simulink model "sx"  (R2015b)
settings: Solver=VariableStepAuto  StartTime=0.0  StopTime=0.003  RelTol=1e-3
settings Model: Creator=hohotulca  LastModifiedBy=hohotulca

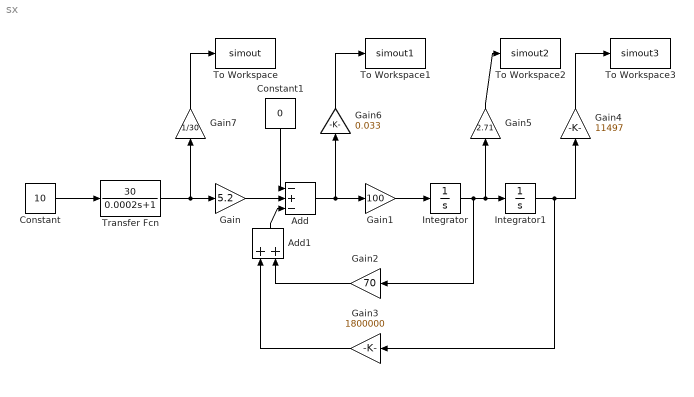
== system sx ==
  Add : Sum  Inputs=-+-
  Add1 : Sum
  Constant : Constant  Value=10
  Constant1 : Constant  Value=0
  Gain : Gain  Gain=5.2
  Gain1 : Gain  Gain=100
  Gain2 : Gain  Gain=70
  Gain3 : Gain  Gain=1800000
  Gain4 : Gain  Gain=11497
  Gain5 : Gain  Gain=2.71
  Gain6 : Gain  Gain=0.033
  Gain7 : Gain  Gain=1/30
  Integrator : Integrator
  Integrator1 : Integrator
  To Workspace : ToWorkspace  VariableName=simout  SaveFormat=Timeseries  SampleTime=-1
  To Workspace1 : ToWorkspace  VariableName=simout1  SaveFormat=Timeseries  SampleTime=-1
  To Workspace2 : ToWorkspace  VariableName=simout2  SaveFormat=Timeseries  SampleTime=-1
  To Workspace3 : ToWorkspace  VariableName=simout3  SaveFormat=Timeseries  SampleTime=-1
  Transfer Fcn : TransferFcn  Numerator=[30]  Denominator=[0.0002 1]
  wires:
  Constant/1 -> Transfer Fcn/1
  Transfer Fcn/1 -> Gain/1, Gain7/1
  Gain/1 -> Add/2
  Add/1 -> Gain1/1, Gain6/1
  Gain1/1 -> Integrator/1
  Integrator/1 -> Gain5/1, Integrator1/1, Gain2/1
  Gain2/1 -> Add1/2
  Add1/1 -> Add/3
  Gain3/1 -> Add1/1
  Integrator1/1 -> Gain3/1, Gain4/1
  Constant1/1 -> Add/1
  Gain7/1 -> To Workspace/1
  Gain6/1 -> To Workspace1/1
  Gain5/1 -> To Workspace2/1
  Gain4/1 -> To Workspace3/1
